simulink model "sampleModel144"  (R2021b)
settings: Solver=VariableStepAuto  StartTime=0.0  StopTime=10.0  RelTol=1e-3
undefined symbols (not defined in the file or in its folder): DiscIntNeverNeededParam, Newton, Raphson
libraries: simulink x15, slpidlib x4
settings Model: Creator=user  LastModifiedBy=user

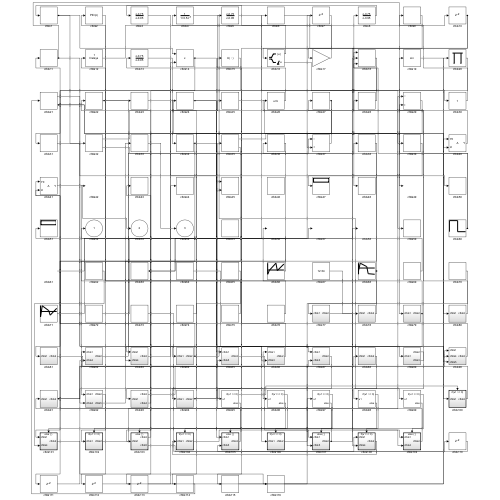
[thumbnail: Simulink's stored preview of the top-level diagram]
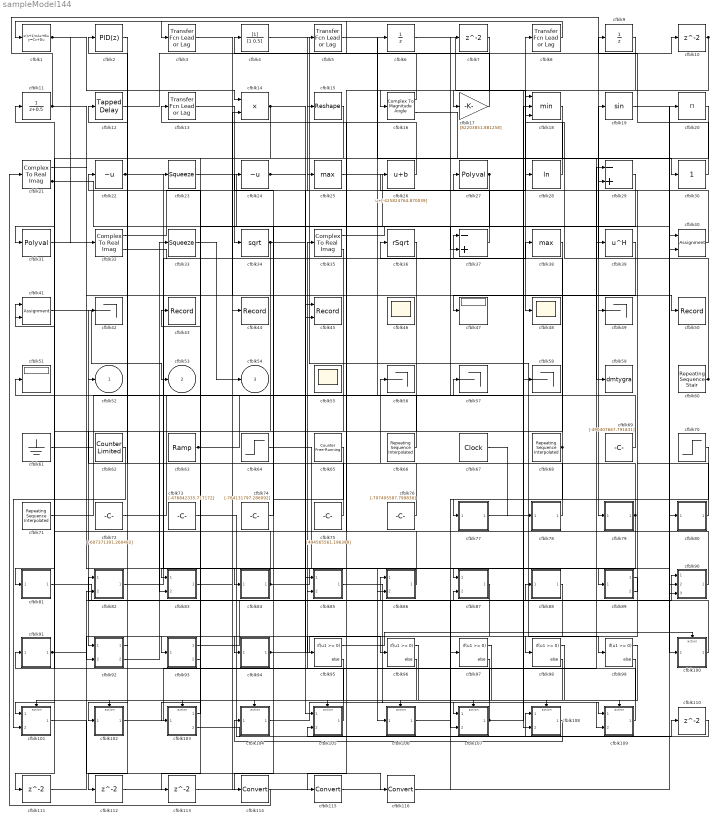
== system sampleModel144 ==
  cfblk1 : DiscreteStateSpace
  cfblk{7,10,110..113} (6 alike) : Delay  SampleTime=1
  cfblk100 : Subsystem  TreatAsAtomicUnit=on
  cfblk101 : Subsystem  TreatAsAtomicUnit=on
  cfblk102 : Subsystem  TreatAsAtomicUnit=on
  cfblk103 : Subsystem  TreatAsAtomicUnit=on
  cfblk104 : Subsystem  TreatAsAtomicUnit=on
  cfblk105 : Subsystem  TreatAsAtomicUnit=on
  cfblk106 : Subsystem  TreatAsAtomicUnit=on
  cfblk107 : Subsystem  TreatAsAtomicUnit=on
  cfblk108 : Subsystem  TreatAsAtomicUnit=on
  cfblk109 : Subsystem  TreatAsAtomicUnit=on
  cfblk11 : DiscreteTransferFcn  SampleTime=1
  cfblk114 : DataTypeConversion
  cfblk115 : DataTypeConversion
  cfblk116 : DataTypeConversion
  cfblk12 : simulink/Discrete/Tapped Delay  vinit=0.0  samptime=-1  NumDelays=1  DelayOrder=Oldest  includeCurrent=off
  cfblk{3,5,8,13} (4 alike) : simulink/Discrete/Transfer Fcn Lead or Lag  PoleZ=0.95  ZeroZ=0.75  ICPrevOutput=0.0  ICPrevInput=0.0  DoSatur=off
      settings: SourceProductBaseCode=SL
  cfblk14 : Product
  cfblk15 : Reshape
  cfblk16 : ComplexToMagnitudeAngle
  cfblk17 : Gain  Gain=[82203851.881258]
  cfblk18 : MinMax  Inputs=3
  cfblk19 : Trigonometry
  cfblk2 : slpidlib/PID Controller  Controller=PID  Form=Parallel  TimeDomain=Discrete-time  UseExternalTs=off  SampleTime=1  IntegratorMethod=Forward Euler  FilterMethod=Forward Euler  ControllerParametersSource=internal  P=1  I=1  D=0  UseFilter=on  N=100  TunerSelectOption=Transfer Function Based (PID Tuner App)  InitialConditionSource=internal  InitialConditionForIntegrator=0  InitialConditionForFilter=0  DifferentiatorICPrevScaledInput=0  ExternalReset=none  TrackingMode=off  Kt=1  LimitOutput=off  SatLimitsSource=internal  UpperSaturationLimit=inf  LowerSaturationLimit=-inf  LinearizeAsGain=off  AntiWindupMode=none  Kb=1  POutMin=[]  POutMax=[]  IOutMin=[]  IOutMax=[]  DOutMin=[]  DOutMax=[]  NOutMin=[]  NOutMax=[]  SumOutMin=[]  SumOutMax=[]  SaturationOutMin=[]  SaturationOutMax=[]  PParamMin=[]  PParamMax=[]  IParamMin=[]  IParamMax=[]  DParamMin=[]  DParamMax=[]  NParamMin=[]  NParamMax=[]  KbParamMin=[]  KbParamMax=[]  KtParamMin=[]  KtParamMax=[]  KbOutMin=[]  KbOutMax=[]  KtOutMin=[]  KtOutMax=[]  IntegratorOutMin=[]  IntegratorOutMax=[]  FilterOutMin=[]  FilterOutMax=[]  SumI1OutMin=[]  SumI1OutMax=[]  SumI2OutMin=[]  SumI2OutMax=[]  SumI3OutMin=[]  SumI3OutMax=[]  SumI4OutMin=[]  SumI4OutMax=[]  SumDOutMin=[]  SumDOutMax=[]  DifferentiatorOutMin=[]  DifferentiatorOutMax=[]  FilterDiffOutCoefMin=[]  FilterDiffOutCoefMax=[]  ReciprocalOutMin=[]  ReciprocalOutMax=[]  SumDenOutMin=[]  SumDenOutMax=[]  SumNumOutMin=[]  SumNumOutMax=[]  DivideOutMin=[]  DivideOutMax=[]  UdiffTsProdOutMin=[]  UdiffTsProdOutMax=[]  NTsProdOutMin=[]  NTsProdOutMax=[]  UintegralTsProdOutMin=[]  UintegralTsProdOutMax=[]  UngainTsProdOutMin=[]  UngainTsProdOutMax=[]  IntegratorContinuousStateAttributes=''  IntegratorStateMustResolveToSignalObject=off  IntegratorRTWStateStorageClass=Auto  FilterContinuousStateAttributes=''  FilterStateMustResolveToSignalObject=off  FilterRTWStateStorageClass=Auto  ParallelPVariant=InternalParameters  IdealPVariant=Disabled  IVariant=InternalParameters  DVariant=InternalParameters  IntegratorVariant=Discrete  SatVariant=Disabled  AWVariant=Passthrough  PCopyVariant=Disabled  TRVariant=Disabled  FdbkBlocksVariant=Forward  IdealPFdbkVariant=Disabled  SatFdbkVariant=Disabled  DerivativeFilterVariant=ForwardEulerFilter  NVariant=InternalParameters  NCopyVariant=Disabled  FilterICVariant=InternalICsFilter  IntegratorICVariant=InternalICs  ExternalResetVariant=Disabled  TRSumVariant=Passthrough  SumFdbkVariant=Disabled  SumVariant=Sum_PID  TsampFilterVariant=InternalTs  TsampNgainVariant=Passthrough  TsampIntegralVariant=Passthrough  ExternalSaturationOutDataTypeStr=Inherit: Same as second input
  cfblk20 : Product  Inputs=*
  cfblk21 : ComplexToRealImag
  cfblk22 : UnaryMinus
  cfblk23 : Squeeze
  cfblk24 : UnaryMinus
  cfblk25 : MinMax  Function=max
  cfblk26 : Bias  Bias=[-425824764.870039]
  cfblk27 : Polyval  Coefs=[ +2.081618890e-019, -1.441693666e-014, +4.719686976e-010, -8.536869453e-006, +1.621573104e-001, -8.087801117e+001 ]
  cfblk28 : Math  Operator=log  SaturateOnIntegerOverflow=on
  cfblk29 : Sum  Inputs=-+
  cfblk30 : simulink/Math Operations/Slider Gain  gain=1  low=0  high=2
  cfblk31 : Polyval  Coefs=[ +2.081618890e-019, -1.441693666e-014, +4.719686976e-010, -8.536869453e-006, +1.621573104e-001, -8.087801117e+001 ]
  cfblk32 : ComplexToRealImag
  cfblk33 : Squeeze
  cfblk34 : Sqrt  SaturateOnIntegerOverflow=on
  cfblk35 : ComplexToRealImag
  cfblk36 : Sqrt  Operator=rSqrt  AlgorithmType=Newton-Raphson  SaturateOnIntegerOverflow=on
  cfblk37 : Sum  Inputs=-+
  cfblk38 : MinMax  Function=max
  cfblk39 : Math  Operator=hermitian  SaturateOnIntegerOverflow=on
  cfblk4 : DiscreteFilter  SampleTime=1
  cfblk40 : Assignment  DiagnosticForDimensions=Warning  IndexOptions=Index vector (dialog)  Indices=1  OutputSizes=1
  cfblk41 : Assignment  DiagnosticForDimensions=Warning  IndexOptions=Index vector (dialog)  Indices=1  OutputSizes=1
  cfblk{42,49,56..58} (5 alike) : Terminator
  cfblk43 : Record  FileSettingsInternal="{\"entries\":[{\"content\":{\"excelSettings\":{\"content\":{},\"type\":\"Streamout.ExcelSettings\"}},\"type\":\"Streamout.FileSettingStorage\",\"uuid\":\"5c4a37b6-0359-467e-84e6-9317a0811d0a\"}],\"packageUris\":[\"http://schema.mathworks.com/mf0/streamout_blocks/R2020a\"],\"version\":\"1.0\"}"  SignalsInternal="{\"entries\":[{\"content\":{\"signals\":[{\"content\":{\"blockPath\":[\"sampleModel144/cfblk43\"],\"channel\":[],\"dimensions\":[1],\"domain\":\"sampleModel144/cfblk43\",\"lineColor\":\"#d95319\",\"plots\":[1],\"port\":1,\"sid\":[\"\"],\"signalID\":5204,\"signalName\":\"cfblk103:1\"},\"type\":\"RecordBlkView.Signal\",\"uuid\":\"9621bb84-a48d-416a-9409-d8cbd1ebf58d\"}]},\"type\":\"RecordBlkView.InputSignals\",\"uuid\":\"23b9c5c9-19cf-4bac-a036-d5d4f1511d02\"}],\"packageUris\":[\"http://schema.mathworks.com/mf0/streamout_blocks/R2020a\"],\"version\":\"1.0\"}"  VisualizationBindings="{\"sparklinesplugin\":{\"info\":[{\"bindingParametersList\":[],\"subplotID\":1}]}}"
  cfblk44 : Record  FileSettingsInternal="{\"entries\":[{\"content\":{\"excelSettings\":{\"content\":{},\"type\":\"Streamout.ExcelSettings\"}},\"type\":\"Streamout.FileSettingStorage\",\"uuid\":\"03f92004-a9d3-4a0e-b80c-98bf6b8b5017\"}],\"packageUris\":[\"http://schema.mathworks.com/mf0/streamout_blocks/R2020a\"],\"version\":\"1.0\"}"  SignalsInternal="{\"entries\":[{\"content\":{\"signals\":[{\"content\":{\"blockPath\":[\"sampleModel144/cfblk44\"],\"channel\":[],\"dimensions\":[1],\"domain\":\"sampleModel144/cfblk44\",\"lineColor\":\"#4dbeee\",\"plots\":[1],\"port\":1,\"sid\":[\"\"],\"signalID\":5220,\"signalName\":\"cfblk71\"},\"type\":\"RecordBlkView.Signal\",\"uuid\":\"c2fc6b42-ec73-41e0-9d10-4ee77b5be672\"}]},\"type\":\"RecordBlkView.InputSignals\",\"uuid\":\"632f383e-e8e8-4e3e-9502-4cccf17acb85\"}],\"packageUris\":[\"http://schema.mathworks.com/mf0/streamout_blocks/R2020a\"],\"version\":\"1.0\"}"  VisualizationBindings="{\"sparklinesplugin\":{\"info\":[{\"bindingParametersList\":[],\"subplotID\":1}]}}"
  cfblk45 : Record  FileSettingsInternal="{\"entries\":[{\"content\":{\"excelSettings\":{\"content\":{},\"type\":\"Streamout.ExcelSettings\"}},\"type\":\"Streamout.FileSettingStorage\",\"uuid\":\"04b73ee6-1f3f-4c79-aaae-0e4c130555b6\"}],\"packageUris\":[\"http://schema.mathworks.com/mf0/streamout_blocks/R2020a\"],\"version\":\"1.0\"}"  Layout=[1 1]  SignalsInternal="{\"entries\":[{\"content\":{\"signals\":[{\"content\":{\"blockPath\":[\"sampleModel144/cfblk45\"],\"channel\":[],\"dimensions\":[1],\"domain\":\"sampleModel144/cfblk45\",\"lineColor\":\"#a2142f\",\"plots\":[1],\"port\":1,\"sid\":[\"\"],\"signalID\":5208,\"signalName\":\"cfblk14\"},\"type\":\"RecordBlkView.Signal\",\"uuid\":\"97cb9547-06cd-434e-bd16-bfd4ee99d097\"},{\"content\":{\"blockPath\":[\"sampleModel144/cfblk45\"],\"channel\":[],\"dimensions\":[1],\"domain\":\"sampleModel144/cfblk45\",\"lineColor\":\"#139fff\",\"plots\":[1],\"port\":2,\"sid\":[\"\"],\"signalID\":5212,\"signalName\":\"cfblk3\"},\"type\":\"RecordBlkView.Signal\",\"uuid\":\"7a9564d6-097e-4b2d-9d37-b1788dcbb395\"}]},\"type\":\"RecordBlkView.InputSignals\",\"uuid\":\"7f23c1a6-79f1-47cc-a483-1563733ee431\"}],\"packageUris\":[\"http://schema.mathworks.com/mf0/streamout_blocks/R2020a\"],\"version\":\"1.0\"}"  VisualizationBindings="{\"xyplotplugin\":{\"info\":[{\"series\":[{\"bindingParametersList\":[{\"parameter\":\"X-Axis\",\"signalID\":5208,\"signalName\":\"cfblk14\"},{\"parameter\":\"Y-Axis\",\"signalID\":5212,\"signalName\":\"cfblk3\"}],\"seriesID\":37859}],\"subplotID\":1}]}}"  CompatibilityTag=XY
  cfblk46 : Scope
      settings: Floating=on
  cfblk47 : Display
  cfblk48 : Scope
  cfblk50 : Record  FileSettingsInternal="{\"entries\":[{\"content\":{\"excelSettings\":{\"content\":{},\"type\":\"Streamout.ExcelSettings\"}},\"type\":\"Streamout.FileSettingStorage\",\"uuid\":\"9c2b4a6c-49af-440e-8358-9805173d7e4c\"}],\"packageUris\":[\"http://schema.mathworks.com/mf0/streamout_blocks/R2020a\"],\"version\":\"1.0\"}"  SignalsInternal="{\"entries\":[{\"content\":{\"signals\":[{\"content\":{\"blockPath\":[\"sampleModel144/cfblk50\"],\"channel\":[],\"dimensions\":[1],\"domain\":\"sampleModel144/cfblk50\",\"lineColor\":\"#77ac30\",\"plots\":[1],\"port\":1,\"sid\":[\"\"],\"signalID\":5216,\"signalName\":\"cfblk11\"},\"type\":\"RecordBlkView.Signal\",\"uuid\":\"50ec43a9-0023-4b49-9f3d-5174647fc26d\"}]},\"type\":\"RecordBlkView.InputSignals\",\"uuid\":\"1b3cebce-2def-4e8e-90ba-a55665d60361\"}],\"packageUris\":[\"http://schema.mathworks.com/mf0/streamout_blocks/R2020a\"],\"version\":\"1.0\"}"  VisualizationBindings="{\"sparklinesplugin\":{\"info\":[{\"bindingParametersList\":[],\"subplotID\":1}]}}"
  cfblk51 : Display
  cfblk55 : Scope
      settings: Floating=on
  cfblk59 : ToWorkspace  VariableName=dmtygra  SaveFormat=Timeseries  SampleTime=-1
  cfblk6 : UnitDelay  HasFrameUpgradeWarning=on
  cfblk60 : simulink/Sources/Repeating Sequence Stair  OutValues=[829001735.314085, 808533127.402397]  tsamp=-1  OutMin=[]  OutMax=[]  OutDataTypeStr=double  OutputDataTypeScalingMode=double  OutDataType=fixdt(0,8)  ConRadixGroup=Best Precision: Vector-wise  OutScaling=2^-12
  cfblk61 : Ground
  cfblk62 : simulink/Sources/Counter Limited  uplimit=[327.000000]  tsamp=-1
  cfblk63 : simulink/Sources/Ramp  slope=[7447.980108]  start=[29.705167]  InitialOutput=[330251.604503]
  cfblk64 : Step  Time=[34.000000]  Before=[375351102.117326]  After=[-26613857.033650]  SampleTime=0
  cfblk65 : simulink/Sources/Counter Free-Running  NumBits=[16.000000]  tsamp=-1
  cfblk66 : simulink/Sources/Repeating Sequence Interpolated  OutValues=[-596507883.427384, -30961132.156261, 983514302.328807, -93919406.075594, 850863097.634730]  TimeValues=[0 0.1 0.5 0.6 1].'  LookUpMeth=Use Input Nearest  tsamp=0.01  OutMin=[]  OutMax=[]  OutDataTypeStr=double  OutputDataTypeScalingMode=double  OutDataType=fixdt(0,8)  OutScaling=2^-10
  cfblk67 : DigitalClock
  cfblk68 : simulink/Sources/Repeating Sequence Interpolated  OutValues=[-355924708.923889, 658030172.948734, 186661830.304645, -770492534.463005, -834534299.027654]  TimeValues=[0 0.1 0.5 0.6 1].'  LookUpMeth=Use Input Nearest  tsamp=0.01  OutMin=[]  OutMax=[]  OutDataTypeStr=double  OutputDataTypeScalingMode=double  OutDataType=fixdt(0,8)  OutScaling=2^-10
  cfblk69 : Constant  Value=[-490407667.791831]  SampleTime=1
  cfblk70 : Step  Time=[49.000000]  Before=[-461429568.151026]  After=[-181712344.934336]  SampleTime=0
  cfblk71 : simulink/Sources/Repeating Sequence Interpolated  OutValues=[-560222174.338453, 578998642.352277, 64467304.021254, -379923535.922782, 322927003.598356]  TimeValues=[0 0.1 0.5 0.6 1].'  LookUpMeth=Interpolation-Use End Values  tsamp=0.01  OutMin=[]  OutMax=[]  OutDataTypeStr=double  OutputDataTypeScalingMode=double  OutDataType=fixdt(0,8)  OutScaling=2^-10
  cfblk72 : Constant  Value=[-607371301.260492]  SampleTime=1
  cfblk73 : Constant  Value=[-476842335.717172]  SampleTime=1
  cfblk74 : Constant  Value=[-764131797.286092]  SampleTime=1
  cfblk75 : Constant  Value=[494565561.196399]  SampleTime=1
  cfblk76 : Constant  Value=[-707405587.799836]  SampleTime=1
  cfblk77 : Subsystem
  cfblk78 : Subsystem
  cfblk79 : Subsystem
  cfblk80 : Subsystem
  cfblk81 : Subsystem
  cfblk82 : Subsystem
  cfblk83 : Subsystem
  cfblk84 : Subsystem
  cfblk85 : Subsystem
  cfblk86 : Subsystem
  cfblk87 : Subsystem
  cfblk88 : Subsystem
  cfblk89 : Subsystem
  cfblk9 : UnitDelay  HasFrameUpgradeWarning=on
  cfblk90 : Subsystem
  cfblk91 : Subsystem
  cfblk92 : Subsystem
  cfblk93 : Subsystem
  cfblk94 : Subsystem
  cfblk{95..99} (5 alike) : If  IfExpression=u1 >= 0  SampleTime=1
  cfblk52 : Outport
  cfblk53 : Outport  Port=2
  cfblk54 : Outport  Port=3
  wires:
  cfblk1/1 -> cfblk32/1, cfblk14/1
  cfblk104/1(cfblk2) -> cfblk109/1(cfblk1)
  cfblk33/1 -> cfblk54/1
  cfblk68/1 -> cfblk36/1, cfblk107/2(cfblk5)
  cfblk73/1 -> cfblk108/1(cfblk1)
  cfblk105/1(cfblk2) -> cfblk91/1(cfblk1)
  cfblk75/1 -> cfblk12/1
  cfblk84/1(cfblk2) -> cfblk87/1(cfblk1), cfblk41/1
  cfblk28/1 -> cfblk8/1
  cfblk66/1 -> cfblk51/1
  cfblk4/1 -> cfblk99/1
  cfblk17/1 -> cfblk1/1
  cfblk13/1 -> cfblk34/1
  cfblk7/1 -> cfblk17/1
  cfblk109/1(cfblk2) -> cfblk35/1
  cfblk81/1(cfblk2) -> cfblk87/2(cfblk3)
  cfblk88/1(cfblk2) -> cfblk93/1(cfblk1)
  cfblk11/1 -> cfblk79/1(cfblk1), cfblk50/1
  cfblk25/1 -> cfblk49/1
  cfblk22/1 -> cfblk84/1(cfblk1), cfblk23/1
  cfblk26/1 -> cfblk13/1
  cfblk67/1 -> cfblk78/1(cfblk1)
  cfblk85/1(cfblk2) -> cfblk107/1(cfblk1)
  cfblk72/1 -> cfblk6/1
  cfblk60/1 -> cfblk19/1, cfblk18/3
  cfblk37/1 -> cfblk26/1
  cfblk6/1 -> cfblk48/1
  cfblk40/1 -> cfblk18/1
  cfblk82/1(cfblk2) -> cfblk37/1
  cfblk93/1(cfblk2) -> cfblk90/1(cfblk1)
  cfblk94/1(cfblk2) -> cfblk96/1, cfblk28/1
  cfblk93/2(cfblk4) -> cfblk22/1
  cfblk8/1 -> cfblk3/1
  cfblk41/1 -> cfblk53/1
  cfblk29/1 -> cfblk37/2
  cfblk15/1 -> cfblk81/1(cfblk1)
  cfblk92/2(cfblk5) -> cfblk33/1
  cfblk108/1(cfblk2) -> cfblk104/1(cfblk1)
  cfblk5/1 -> cfblk30/1
  cfblk32/1 -> cfblk5/1
  cfblk23/1 -> cfblk59/1
  cfblk76/1 -> cfblk2/1
  cfblk31/1 -> cfblk89/1(cfblk1)
  cfblk107/1(cfblk2) -> cfblk58/1, cfblk41/2
  cfblk30/1 -> cfblk9/1
  cfblk35/1 -> cfblk40/2
  cfblk78/1(cfblk2) -> cfblk42/1
  cfblk36/1 -> cfblk92/1(cfblk1)
  cfblk106/1(cfblk2) -> cfblk88/1(cfblk1)
  cfblk102/1(cfblk2) -> cfblk29/1
  cfblk39/1 -> cfblk47/1
  cfblk83/1(cfblk2) -> cfblk25/1
  cfblk38/1 -> cfblk101/1(cfblk1)
  cfblk71/1 -> cfblk44/1
  cfblk87/1(cfblk2) -> cfblk92/2(cfblk4)
  cfblk61/1 -> cfblk7/1
  cfblk34/1 -> cfblk105/1(cfblk1), cfblk83/2(cfblk4)
  cfblk77/1(cfblk2) -> cfblk109/2(cfblk4)
  cfblk21/1 -> cfblk90/2(cfblk4)
  cfblk9/1 -> cfblk95/1
  cfblk10/1 -> cfblk16/1, cfblk108/2(cfblk4)
  cfblk19/1 -> cfblk80/1(cfblk1)
  cfblk27/1 -> cfblk94/1(cfblk1), cfblk113/1
  cfblk89/1(cfblk2) -> cfblk98/1
  cfblk24/1 -> cfblk90/3(cfblk5), cfblk86/2(cfblk3)
  cfblk62/1 -> cfblk101/2(cfblk4)
  cfblk14/1 -> cfblk45/1, cfblk31/1
  cfblk64/1 -> cfblk106/1(cfblk1)
  cfblk89/2(cfblk3) -> cfblk27/1
  cfblk12/1 -> cfblk10/1
  cfblk70/1 -> cfblk77/1(cfblk1)
  cfblk18/1 -> cfblk103/1(cfblk1)
  cfblk86/1(cfblk2) -> cfblk15/1
  cfblk80/1(cfblk2) -> cfblk29/2
  cfblk74/1 -> cfblk24/1
  cfblk63/1 -> cfblk57/1, cfblk18/2
  cfblk32/2 -> cfblk38/1
  cfblk90/1(cfblk2) -> cfblk11/1
  cfblk21/2 -> cfblk85/1(cfblk1), cfblk100/1(cfblk1)
  cfblk69/1 -> cfblk52/1
  cfblk16/1 -> cfblk4/1
  cfblk103/1(cfblk2) -> cfblk43/1
  cfblk16/2 -> cfblk39/1
  cfblk3/1 -> cfblk45/2
  cfblk100/1(cfblk2) -> cfblk82/1(cfblk1)
  cfblk91/1(cfblk2) -> cfblk85/2(cfblk5), cfblk86/1(cfblk1)
  cfblk2/1 -> cfblk102/1(cfblk1)
  cfblk79/1(cfblk2) -> cfblk83/1(cfblk1), cfblk56/1
  cfblk95/1 -> cfblk100/Action
  cfblk95/2 -> cfblk101/Action
  cfblk96/1 -> cfblk102/Action
  cfblk96/2 -> cfblk103/Action
  cfblk97/1 -> cfblk104/Action
  cfblk97/2 -> cfblk105/Action
  cfblk98/1 -> cfblk106/Action
  cfblk98/2 -> cfblk107/Action
  cfblk99/1 -> cfblk108/Action
  cfblk99/2 -> cfblk109/Action
  cfblk103/2(cfblk5) -> cfblk110/1
  cfblk110/1 -> cfblk105/2(cfblk5)
  cfblk35/2 -> cfblk111/1
  cfblk111/1 -> cfblk82/2(cfblk4)
  cfblk92/1(cfblk2) -> cfblk112/1
  cfblk112/1 -> cfblk97/1
  cfblk113/1 -> cfblk14/2
  cfblk65/1 -> cfblk114/1
  cfblk114/1 -> cfblk21/1
  cfblk20/1 -> cfblk115/1
  cfblk115/1 -> cfblk40/1
  cfblk101/1(cfblk2) -> cfblk116/1
  cfblk116/1 -> cfblk20/1

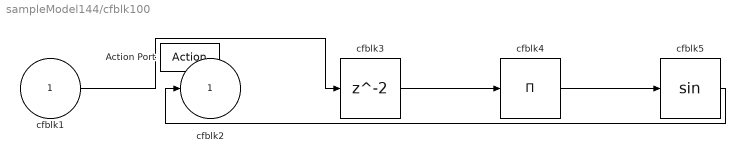
== system sampleModel144/cfblk100 ==
  cfblk1 : Inport
  Action Port : ActionPort  ActionPortLabel=if(u1 >= 0)
  cfblk3 : Delay
  cfblk4 : Product  Inputs=*
  cfblk5 : Trigonometry
  cfblk2 : Outport
  wires:
  cfblk3/1 -> cfblk4/1
  cfblk4/1 -> cfblk5/1
  cfblk5/1 -> cfblk2/1
  cfblk1/1 -> cfblk3/1

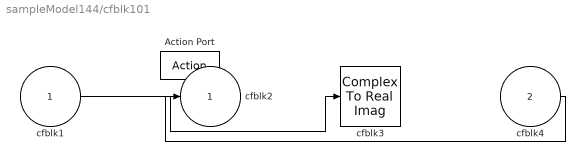
== system sampleModel144/cfblk101 ==
  cfblk1 : Inport
  cfblk4 : Inport  Port=2
  Action Port : ActionPort  ActionPortLabel=else
  cfblk3 : ComplexToRealImag
  cfblk2 : Outport
  wires:
  cfblk1/1 -> cfblk3/1
  cfblk4/1 -> cfblk2/1

== system sampleModel144/cfblk102 ==
  cfblk1 : Inport
  Action Port : ActionPort  ActionPortLabel=if(u1 >= 0)
  cfblk3 : DiscreteTransferFcn
  cfblk2 : Outport
  wires:
  cfblk3/1 -> cfblk2/1
  cfblk1/1 -> cfblk3/1

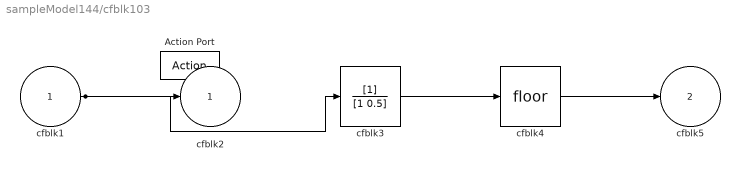
== system sampleModel144/cfblk103 ==
  cfblk1 : Inport
  Action Port : ActionPort  ActionPortLabel=else
  cfblk3 : DiscreteFilter
  cfblk4 : Rounding
  cfblk2 : Outport
  cfblk5 : Outport  Port=2
  wires:
  cfblk1/1 -> cfblk3/1, cfblk2/1
  cfblk4/1 -> cfblk5/1
  cfblk3/1 -> cfblk4/1

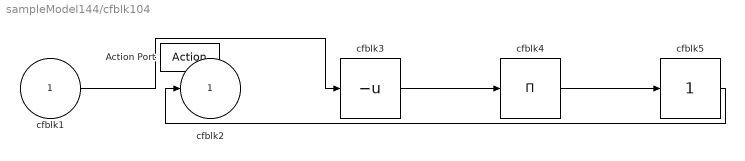
== system sampleModel144/cfblk104 ==
  cfblk1 : Inport
  Action Port : ActionPort  ActionPortLabel=if(u1 >= 0)
  cfblk3 : UnaryMinus
  cfblk4 : Product  Inputs=*
  cfblk5 : simulink/Math Operations/Slider Gain  gain=1  low=0  high=2
  cfblk2 : Outport
  wires:
  cfblk3/1 -> cfblk4/1
  cfblk5/1 -> cfblk2/1
  cfblk1/1 -> cfblk3/1
  cfblk4/1 -> cfblk5/1

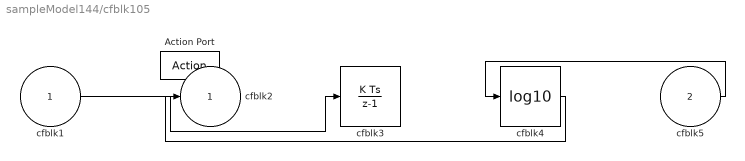
== system sampleModel144/cfblk105 ==
  cfblk1 : Inport
  cfblk5 : Inport  Port=2
  Action Port : ActionPort  ActionPortLabel=else
  cfblk3 : DiscreteIntegrator  SampleTime=-1  ICPrevOutput=DiscIntNeverNeededParam  ICPrevScaledInput=DiscIntNeverNeededParam
  cfblk4 : Math  Operator=log10  SaturateOnIntegerOverflow=on
  cfblk2 : Outport
  wires:
  cfblk5/1 -> cfblk4/1
  cfblk1/1 -> cfblk3/1
  cfblk4/1 -> cfblk2/1

== system sampleModel144/cfblk106 ==
  cfblk1 : Inport
  Action Port : ActionPort  ActionPortLabel=if(u1 >= 0)
  cfblk3 : simulink/Math Operations/MinMax Running Resettable  Function=min  vinit=0.0
  cfblk2 : Outport
  wires:
  cfblk1/1 -> cfblk3/1, cfblk3/2
  cfblk3/1 -> cfblk2/1

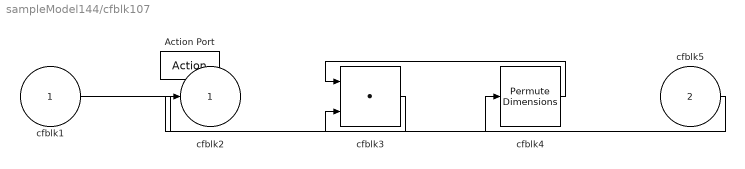
== system sampleModel144/cfblk107 ==
  cfblk1 : Inport
  cfblk5 : Inport  Port=2
  Action Port : ActionPort  ActionPortLabel=else
  cfblk3 : DotProduct  InputSameDT=on  OutDataTypeStr=Inherit: Inherit via internal rule
  cfblk4 : PermuteDimensions
  cfblk2 : Outport
  wires:
  cfblk4/1 -> cfblk3/1
  cfblk5/1 -> cfblk3/2
  cfblk1/1 -> cfblk4/1
  cfblk3/1 -> cfblk2/1

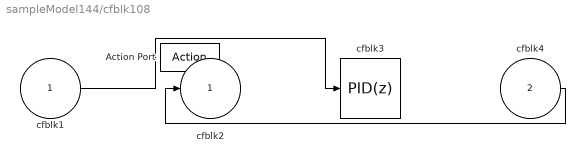
== system sampleModel144/cfblk108 ==
  cfblk1 : Inport
  cfblk4 : Inport  Port=2
  Action Port : ActionPort  ActionPortLabel=if(u1 >= 0)
  cfblk3 : slpidlib/PID Controller  Controller=PID  Form=Parallel  TimeDomain=Discrete-time  UseExternalTs=off  SampleTime=-1  IntegratorMethod=Forward Euler  FilterMethod=Forward Euler  ControllerParametersSource=internal  P=1  I=1  D=0  UseFilter=on  N=100  TunerSelectOption=Transfer Function Based (PID Tuner App)  InitialConditionSource=internal  InitialConditionForIntegrator=0  InitialConditionForFilter=0  DifferentiatorICPrevScaledInput=0  ExternalReset=none  TrackingMode=off  Kt=1  LimitOutput=off  SatLimitsSource=internal  UpperSaturationLimit=inf  LowerSaturationLimit=-inf  LinearizeAsGain=off  AntiWindupMode=none  Kb=1  POutMin=[]  POutMax=[]  IOutMin=[]  IOutMax=[]  DOutMin=[]  DOutMax=[]  NOutMin=[]  NOutMax=[]  SumOutMin=[]  SumOutMax=[]  SaturationOutMin=[]  SaturationOutMax=[]  PParamMin=[]  PParamMax=[]  IParamMin=[]  IParamMax=[]  DParamMin=[]  DParamMax=[]  NParamMin=[]  NParamMax=[]  KbParamMin=[]  KbParamMax=[]  KtParamMin=[]  KtParamMax=[]  KbOutMin=[]  KbOutMax=[]  KtOutMin=[]  KtOutMax=[]  IntegratorOutMin=[]  IntegratorOutMax=[]  FilterOutMin=[]  FilterOutMax=[]  SumI1OutMin=[]  SumI1OutMax=[]  SumI2OutMin=[]  SumI2OutMax=[]  SumI3OutMin=[]  SumI3OutMax=[]  SumI4OutMin=[]  SumI4OutMax=[]  SumDOutMin=[]  SumDOutMax=[]  DifferentiatorOutMin=[]  DifferentiatorOutMax=[]  FilterDiffOutCoefMin=[]  FilterDiffOutCoefMax=[]  ReciprocalOutMin=[]  ReciprocalOutMax=[]  SumDenOutMin=[]  SumDenOutMax=[]  SumNumOutMin=[]  SumNumOutMax=[]  DivideOutMin=[]  DivideOutMax=[]  UdiffTsProdOutMin=[]  UdiffTsProdOutMax=[]  NTsProdOutMin=[]  NTsProdOutMax=[]  UintegralTsProdOutMin=[]  UintegralTsProdOutMax=[]  UngainTsProdOutMin=[]  UngainTsProdOutMax=[]  IntegratorContinuousStateAttributes=''  IntegratorStateMustResolveToSignalObject=off  IntegratorRTWStateStorageClass=Auto  FilterContinuousStateAttributes=''  FilterStateMustResolveToSignalObject=off  FilterRTWStateStorageClass=Auto  ParallelPVariant=InternalParameters  IdealPVariant=Disabled  IVariant=InternalParameters  DVariant=InternalParameters  IntegratorVariant=Discrete  SatVariant=Disabled  AWVariant=Passthrough  PCopyVariant=Disabled  TRVariant=Disabled  FdbkBlocksVariant=Forward  IdealPFdbkVariant=Disabled  SatFdbkVariant=Disabled  DerivativeFilterVariant=ForwardEulerFilter  NVariant=InternalParameters  NCopyVariant=Disabled  FilterICVariant=InternalICsFilter  IntegratorICVariant=InternalICs  ExternalResetVariant=Disabled  TRSumVariant=Passthrough  SumFdbkVariant=Disabled  SumVariant=Sum_PID  TsampFilterVariant=InternalTs  TsampNgainVariant=Passthrough  TsampIntegralVariant=Passthrough  ExternalSaturationOutDataTypeStr=Inherit: Same as second input
  cfblk2 : Outport
  wires:
  cfblk4/1 -> cfblk2/1
  cfblk1/1 -> cfblk3/1

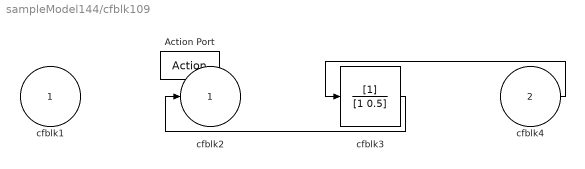
== system sampleModel144/cfblk109 ==
  cfblk1 : Inport
  cfblk4 : Inport  Port=2
  Action Port : ActionPort  ActionPortLabel=else
  cfblk3 : DiscreteFilter
  cfblk2 : Outport
  wires:
  cfblk3/1 -> cfblk2/1
  cfblk4/1 -> cfblk3/1

== system sampleModel144/cfblk77 ==
  cfblk1 : Inport
  cfblk3 : Trigonometry
  cfblk2 : Outport
  wires:
  cfblk1/1 -> cfblk2/1, cfblk3/1

== system sampleModel144/cfblk78 ==
  cfblk1 : Inport
  cfblk3 : DiscreteStateSpace
  cfblk2 : Outport
  wires:
  cfblk3/1 -> cfblk2/1
  cfblk1/1 -> cfblk3/1

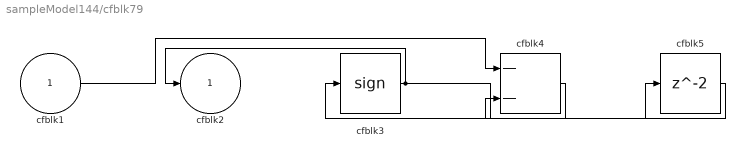
== system sampleModel144/cfblk79 ==
  cfblk1 : Inport
  cfblk3 : Signum
  cfblk4 : Sum  Inputs=--
  cfblk5 : Delay  SampleTime=1
  cfblk2 : Outport
  wires:
  cfblk3/1 -> cfblk2/1, cfblk5/1
  cfblk1/1 -> cfblk4/1
  cfblk4/1 -> cfblk3/1
  cfblk5/1 -> cfblk4/2

== system sampleModel144/cfblk80 ==
  cfblk1 : Inport
  cfblk3 : Product  Inputs=*
  cfblk2 : Outport
  wires:
  cfblk1/1 -> cfblk3/1
  cfblk3/1 -> cfblk2/1

== system sampleModel144/cfblk81 ==
  cfblk1 : Inport
  cfblk3 : slpidlib/PID Controller (2DOF)  Controller=PID  Form=Parallel  TimeDomain=Discrete-time  UseExternalTs=off  SampleTime=1  IntegratorMethod=Forward Euler  FilterMethod=Forward Euler  ControllerParametersSource=internal  P=1  I=1  D=0  UseFilter=on  N=100  b=1  c=1  TunerSelectOption=Transfer Function Based (PID Tuner App)  InitialConditionSource=internal  InitialConditionForIntegrator=0  InitialConditionForFilter=0  DifferentiatorICPrevScaledInput=0  ExternalReset=none  TrackingMode=off  Kt=1  LimitOutput=off  SatLimitsSource=internal  UpperSaturationLimit=inf  LowerSaturationLimit=-inf  LinearizeAsGain=off  AntiWindupMode=none  Kb=1  POutMin=[]  POutMax=[]  IOutMin=[]  IOutMax=[]  DOutMin=[]  DOutMax=[]  NOutMin=[]  NOutMax=[]  bOutMin=[]  bOutMax=[]  cOutMin=[]  cOutMax=[]  SumOutMin=[]  SumOutMax=[]  SaturationOutMin=[]  SaturationOutMax=[]  PParamMin=[]  PParamMax=[]  IParamMin=[]  IParamMax=[]  DParamMin=[]  DParamMax=[]  NParamMin=[]  NParamMax=[]  bParamMin=[]  bParamMax=[]  cParamMin=[]  cParamMax=[]  KbParamMin=[]  KbParamMax=[]  KtParamMin=[]  KtParamMax=[]  KbOutMin=[]  KbOutMax=[]  KtOutMin=[]  KtOutMax=[]  IntegratorOutMin=[]  IntegratorOutMax=[]  FilterOutMin=[]  FilterOutMax=[]  SumI1OutMin=[]  SumI1OutMax=[]  SumI2OutMin=[]  SumI2OutMax=[]  SumI3OutMin=[]  SumI3OutMax=[]  SumI4OutMin=[]  SumI4OutMax=[]  SumDOutMin=[]  SumDOutMax=[]  Sum1OutMin=[]  Sum1OutMax=[]  Sum2OutMin=[]  Sum2OutMax=[]  Sum3OutMin=[]  Sum3OutMax=[]  DifferentiatorOutMin=[]  DifferentiatorOutMax=[]  FilterDiffOutCoefMin=[]  FilterDiffOutCoefMax=[]  ReciprocalOutMin=[]  ReciprocalOutMax=[]  SumDenOutMin=[]  SumDenOutMax=[]  SumNumOutMin=[]  SumNumOutMax=[]  DivideOutMin=[]  DivideOutMax=[]  UdiffTsProdOutMin=[]  UdiffTsProdOutMax=[]  NTsProdOutMin=[]  NTsProdOutMax=[]  UintegralTsProdOutMin=[]  UintegralTsProdOutMax=[]  UngainTsProdOutMin=[]  UngainTsProdOutMax=[]  IntegratorContinuousStateAttributes=''  IntegratorStateMustResolveToSignalObject=off  IntegratorRTWStateStorageClass=Auto  FilterContinuousStateAttributes=''  FilterStateMustResolveToSignalObject=off  FilterRTWStateStorageClass=Auto  ParallelPVariant=InternalParameters  IdealPVariant=Disabled  IVariant=InternalParameters  DVariant=InternalParameters  bVariant=InternalParameters  cVariant=InternalParameters  IntegratorVariant=Discrete  SatVariant=Disabled  AWVariant=Passthrough  PCopyVariant=Disabled  TRVariant=Disabled  FdbkBlocksVariant=Forward  IdealPFdbkVariant=Disabled  SatFdbkVariant=Disabled  DerivativeFilterVariant=ForwardEulerFilter  NVariant=InternalParameters  NCopyVariant=Disabled  FilterICVariant=InternalICsFilter  IntegratorICVariant=InternalICs  ExternalResetVariant=Disabled  TRSumVariant=Passthrough  SumFdbkVariant=Disabled  SumVariant=Sum_PID  TsampFilterVariant=InternalTs  TsampNgainVariant=Passthrough  TsampIntegralVariant=Passthrough  ExternalSaturationOutDataTypeStr=Inherit: Same as second input
      settings: SourceProductBaseCode=SL
  cfblk2 : Outport
  wires:
  cfblk3/1 -> cfblk2/1
  cfblk1/1 -> cfblk3/1, cfblk3/2

== system sampleModel144/cfblk82 ==
  cfblk1 : Inport
  cfblk4 : Inport  Port=2
  cfblk3 : Constant  Value=[-183573215.800943]  SampleTime=1
  cfblk2 : Outport
  wires:
  cfblk1/1 -> cfblk2/1

== system sampleModel144/cfblk83 ==
  cfblk1 : Inport
  cfblk4 : Inport  Port=2
  cfblk3 : DiscreteZeroPole  Poles=[0 0.5]  Gain=1
  cfblk2 : Outport
  wires:
  cfblk1/1 -> cfblk2/1
  cfblk4/1 -> cfblk3/1

== system sampleModel144/cfblk84 ==
  cfblk1 : Inport
  cfblk3 : PermuteDimensions
  cfblk2 : Outport
  wires:
  cfblk3/1 -> cfblk2/1
  cfblk1/1 -> cfblk3/1

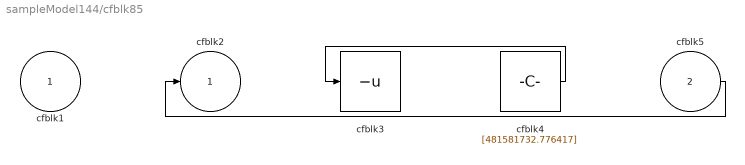
== system sampleModel144/cfblk85 ==
  cfblk1 : Inport
  cfblk5 : Inport  Port=2
  cfblk3 : UnaryMinus
  cfblk4 : Constant  Value=[481581732.776417]  SampleTime=1
  cfblk2 : Outport
  wires:
  cfblk4/1 -> cfblk3/1
  cfblk5/1 -> cfblk2/1

== system sampleModel144/cfblk86 ==
  cfblk1 : Inport
  cfblk3 : Inport  Port=2
  cfblk2 : Outport
  wires:
  cfblk1/1 -> cfblk2/1

== system sampleModel144/cfblk87 ==
  cfblk1 : Inport
  cfblk3 : Inport  Port=2
  cfblk2 : Outport
  wires:
  cfblk1/1 -> cfblk2/1

== system sampleModel144/cfblk88 ==
  cfblk1 : Inport
  cfblk3 : Bias  Bias=[-916073872.083986]
  cfblk2 : Outport
  wires:
  cfblk1/1 -> cfblk3/1
  cfblk3/1 -> cfblk2/1

== system sampleModel144/cfblk89 ==
  cfblk1 : Inport
  cfblk2 : Outport
  cfblk3 : Outport  Port=2
  wires:
  cfblk1/1 -> cfblk3/1, cfblk2/1

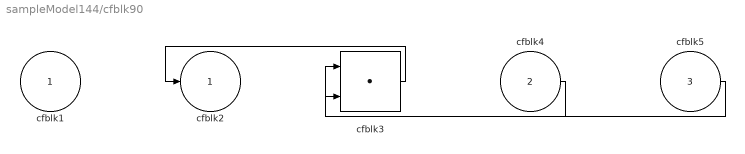
== system sampleModel144/cfblk90 ==
  cfblk1 : Inport
  cfblk4 : Inport  Port=2
  cfblk5 : Inport  Port=3
  cfblk3 : DotProduct  InputSameDT=on  OutDataTypeStr=Inherit: Inherit via internal rule
  cfblk2 : Outport
  wires:
  cfblk3/1 -> cfblk2/1
  cfblk4/1 -> cfblk3/1
  cfblk5/1 -> cfblk3/2

== system sampleModel144/cfblk91 ==
  cfblk1 : Inport
  cfblk3 : Sum  Inputs=|++
  cfblk2 : Outport
  wires:
  cfblk3/1 -> cfblk2/1
  cfblk1/1 -> cfblk3/1, cfblk3/2

== system sampleModel144/cfblk92 ==
  cfblk1 : Inport
  cfblk4 : Inport  Port=2
  cfblk3 : slpidlib/PID Controller (2DOF)  Controller=PID  Form=Parallel  TimeDomain=Discrete-time  UseExternalTs=off  SampleTime=1  IntegratorMethod=Forward Euler  FilterMethod=Forward Euler  ControllerParametersSource=internal  P=1  I=1  D=0  UseFilter=on  N=100  b=1  c=1  TunerSelectOption=Transfer Function Based (PID Tuner App)  InitialConditionSource=internal  InitialConditionForIntegrator=0  InitialConditionForFilter=0  DifferentiatorICPrevScaledInput=0  ExternalReset=none  TrackingMode=off  Kt=1  LimitOutput=off  SatLimitsSource=internal  UpperSaturationLimit=inf  LowerSaturationLimit=-inf  LinearizeAsGain=off  AntiWindupMode=none  Kb=1  POutMin=[]  POutMax=[]  IOutMin=[]  IOutMax=[]  DOutMin=[]  DOutMax=[]  NOutMin=[]  NOutMax=[]  bOutMin=[]  bOutMax=[]  cOutMin=[]  cOutMax=[]  SumOutMin=[]  SumOutMax=[]  SaturationOutMin=[]  SaturationOutMax=[]  PParamMin=[]  PParamMax=[]  IParamMin=[]  IParamMax=[]  DParamMin=[]  DParamMax=[]  NParamMin=[]  NParamMax=[]  bParamMin=[]  bParamMax=[]  cParamMin=[]  cParamMax=[]  KbParamMin=[]  KbParamMax=[]  KtParamMin=[]  KtParamMax=[]  KbOutMin=[]  KbOutMax=[]  KtOutMin=[]  KtOutMax=[]  IntegratorOutMin=[]  IntegratorOutMax=[]  FilterOutMin=[]  FilterOutMax=[]  SumI1OutMin=[]  SumI1OutMax=[]  SumI2OutMin=[]  SumI2OutMax=[]  SumI3OutMin=[]  SumI3OutMax=[]  SumI4OutMin=[]  SumI4OutMax=[]  SumDOutMin=[]  SumDOutMax=[]  Sum1OutMin=[]  Sum1OutMax=[]  Sum2OutMin=[]  Sum2OutMax=[]  Sum3OutMin=[]  Sum3OutMax=[]  DifferentiatorOutMin=[]  DifferentiatorOutMax=[]  FilterDiffOutCoefMin=[]  FilterDiffOutCoefMax=[]  ReciprocalOutMin=[]  ReciprocalOutMax=[]  SumDenOutMin=[]  SumDenOutMax=[]  SumNumOutMin=[]  SumNumOutMax=[]  DivideOutMin=[]  DivideOutMax=[]  UdiffTsProdOutMin=[]  UdiffTsProdOutMax=[]  NTsProdOutMin=[]  NTsProdOutMax=[]  UintegralTsProdOutMin=[]  UintegralTsProdOutMax=[]  UngainTsProdOutMin=[]  UngainTsProdOutMax=[]  IntegratorContinuousStateAttributes=''  IntegratorStateMustResolveToSignalObject=off  IntegratorRTWStateStorageClass=Auto  FilterContinuousStateAttributes=''  FilterStateMustResolveToSignalObject=off  FilterRTWStateStorageClass=Auto  ParallelPVariant=InternalParameters  IdealPVariant=Disabled  IVariant=InternalParameters  DVariant=InternalParameters  bVariant=InternalParameters  cVariant=InternalParameters  IntegratorVariant=Discrete  SatVariant=Disabled  AWVariant=Passthrough  PCopyVariant=Disabled  TRVariant=Disabled  FdbkBlocksVariant=Forward  IdealPFdbkVariant=Disabled  SatFdbkVariant=Disabled  DerivativeFilterVariant=ForwardEulerFilter  NVariant=InternalParameters  NCopyVariant=Disabled  FilterICVariant=InternalICsFilter  IntegratorICVariant=InternalICs  ExternalResetVariant=Disabled  TRSumVariant=Passthrough  SumFdbkVariant=Disabled  SumVariant=Sum_PID  TsampFilterVariant=InternalTs  TsampNgainVariant=Passthrough  TsampIntegralVariant=Passthrough  ExternalSaturationOutDataTypeStr=Inherit: Same as second input
      settings: SourceProductBaseCode=SL
  cfblk2 : Outport
  cfblk5 : Outport  Port=2
  wires:
  cfblk1/1 -> cfblk2/1, cfblk3/1
  cfblk4/1 -> cfblk5/1, cfblk3/2

== system sampleModel144/cfblk93 ==
  cfblk1 : Inport
  cfblk3 : Constant  Value=[842943344.214737]  SampleTime=1
  cfblk2 : Outport
  cfblk4 : Outport  Port=2
  wires:
  cfblk1/1 -> cfblk2/1
  cfblk3/1 -> cfblk4/1

== system sampleModel144/cfblk94 ==
  cfblk1 : Inport
  cfblk3 : DiscreteZeroPole  Poles=[0 0.5]  Gain=1
  cfblk2 : Outport
  wires:
  cfblk1/1 -> cfblk3/1
  cfblk3/1 -> cfblk2/1
